simulink model "speedconversion"  (R2016b)
settings: Solver=VariableStepAuto  StartTime=0.0  StopTime=10.0  RelTol=1e-3
settings Model: Creator=karanverma  LastModifiedBy=karanverma

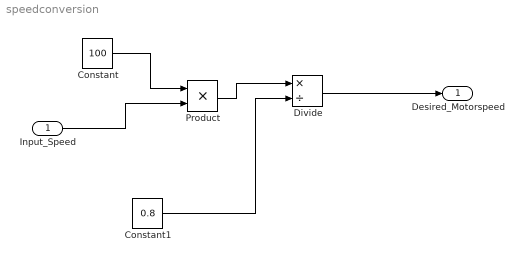
== system speedconversion ==
  Input_Speed : Inport
  Constant : Constant  Value=100
  Constant1 : Constant  Value=0.8
  Divide : Product  Inputs=*/
  Product : Product
  Desired_Motorspeed : Outport
  wires:
  Input_Speed/1 -> Product/2
  Constant/1 -> Product/1
  Constant1/1 -> Divide/2
  Product/1 -> Divide/1
  Divide/1 -> Desired_Motorspeed/1
